simulink model "Quad_att_control"  (R2022b)
settings: Solver=ode4  StartTime=0.0  StopTime=100  FixedStep=0.001  RelTol=1e-3  EnableMultiTasking=on
model workspace (MAT data in the model file):
  A_m = [0  0  0  1  0  0; 0  0  0  0  1  0; 0  0  0  0  0  1; 0  0  0  0  1  1; 0  0  0  1  0  1; 0  0  0  1  1  0]
  A_r = [0  0  0  1  0  0; 0  0  0  0  1  0; 0  0  0  0  0  1; -1  0  0  -6  0  0; 0  -1  0  0  -6  0; 0  0  -1  0  0  -6]
  B_m = [0  0  0; 0  0  0; 0  0  0; 1  0  0; 0  1  0; 0  0  1]
  B_r = [0  0  0; 0  0  0; 0  0  0; 1  0  0; 0  1  0; 0  0  1]
  W_n = 2
  Zeta = 1.5
undefined symbols (not defined in the file): d2r, params, r2d
libraries: slpidlib x3, sharedtransform x2, matrix_library x2, sharedutil x2, uavutilslib x2, slctrlblks x1
settings Model: SimulationMode=accelerator  ParameterArgumentNames=A_r,Zeta  Creator=dsai9  LastModifiedBy=dsai9
settings SolverCC: PositivePriorityOrder=on
settings OptimizationCC: EnhancedBackFolding=on  PassReuseOutputArgsAs=Individual arguments  ZeroExternalMemoryAtStartup=off  ZeroInternalMemoryAtStartup=off  MaxStackSize=64  OptimizeBlockOrder=speed  DifferentSizesBufferReuse=on  OptimizationCustomize=off  EfficientTunableParamExpr=on
settings DebuggingCC: ParameterTunabilityLossMsg=error
settings HardwareCC: ProdBitPerPointer=32  ProdBitPerSizeT=32  ProdBitPerPtrDiffT=32  ProdLargestAtomicInteger=Long  ProdLargestAtomicFloat=Double  ProdWordSize=32  ProdLongLongMode=on  ProdHWDeviceType=ARM Compatible->ARM Cortex
settings RTWCC: Description=Embedded Coder  SystemTargetFile=ert.tlc  HardwareBoard=Raspberry Pi  TLCOptions="-aInlineSetEventsForThisBaseRateFcn=TLC_FALSE -aSuppressMultiTaskScheduler=TLC_FALSE  -aRateBasedStepFcn=0"  TemplateMakefile=ert_default_tmf  Toolchain=GNU GCC Embedded Linux  BuildConfiguration=Faster Runs
settings CodeAppCC: ForceParamTrailComments=on  IgnoreCustomStorageClasses=off  OperatorAnnotations=on  SimulinkDataObjDesc=on  SFDataObjDesc=on  InsertBlockDesc=on
settings ERTTargetCC: SupportVariableSizeSignals=on  ExtModeTransport=2  ExtModeStaticAlloc=on  ExtModeMexFile=ext_xcp  ExtModeIntrfLevel=Level2 - Open

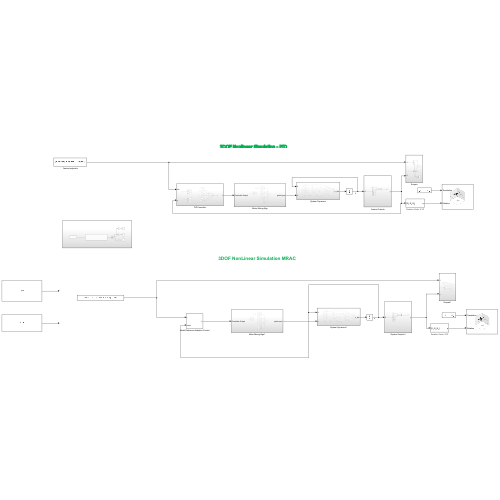
[thumbnail: Simulink's stored preview of the top-level diagram]
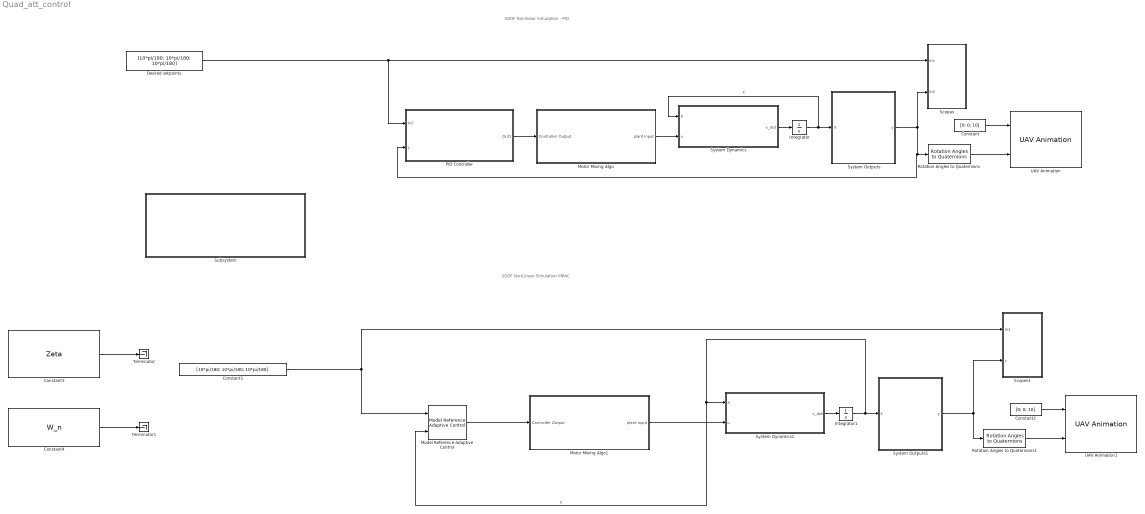
== system Quad_att_control ==
  note: 3DOF NonLinear Simulation MRAC
  note: 3DOF Nonlinear Simulation - PID
  Constant : Constant  Value=[0; 0; 10]
  Constant1 : Constant  Value=[10*pi/180; 10*pi/180; 10*pi/180]
  Constant2 : Constant  Value=[0; 0; 10]
  Constant3 : Constant  Value=Zeta
  Constant4 : Constant  Value=W_n
  Desired setpoints : Constant  Value=[10*pi/180; 10*pi/180; 10*pi/180]
  Integrator : Integrator  InitialCondition=[0;0;0;0;0;0]
  Integrator1 : Integrator  InitialCondition=[0;0;0;0;0;0]
  Model Reference Adaptive Control : slctrlblks/Model Reference Adaptive Control  selectType=Direct  A=A_m  B=B_m  Ahat=0  ALrEnable=on  gamma_a=1  ALrEnableMod=on  Bhat=1  BLrEnable=on  gamma_b=1  BLrEnableMod=on  externalKtauEnable=off  k_tau=-1  estParamOutput=off  Am=A_r  Bm=B_r  kx=0  FBLrEnable=on  gamma_kx=200  FBLrEnableMod=off  kr=0  FFLrEnable=on  gamma_kr=200  FFLrEnableMod=off  AdaptEnable=off  gamma=1  WLrEnableMod=on  Q=1  FeatureTypeOptions=State  nCen=20  cSpanMin=-1  cSpanMax=1  cSig=5  adaptiveCntrlOutport=off  modChoice=None  sigma_val=0.1
  Motor Mixing Algo : Subsystem
  Motor Mixing Algo1 : Subsystem
  PID Controller : Subsystem
  Rotation Angles to Quaternions : sharedtransform/Rotation Angles to Quaternions  rotationOrder=XYZ  aMode=aMode
  Rotation Angles to Quaternions1 : sharedtransform/Rotation Angles to Quaternions  rotationOrder=XYZ  aMode=aMode
  Scopes : Subsystem
  Scopes1 : Subsystem
  Subsystem : Subsystem
  System Dynamics : Subsystem
  System Dynamics1 : Subsystem
  System Outputs : Subsystem
  System Outputs1 : Subsystem
  Terminator : Terminator
  Terminator1 : Terminator
  UAV Animation : uavutilslib/UAV Animation  UAVType=Multirotor  UAVSize=1  InertialZDirection=Down  SampleTime=-1
  UAV Animation1 : uavutilslib/UAV Animation  UAVType=Multirotor  UAVSize=1  InertialZDirection=Down  SampleTime=-1
  wires:
  System Dynamics/1(x_dot) -> Integrator/1
  Integrator/1 -> System Dynamics/1(X), System Outputs/1(X)  "X"
  Motor Mixing Algo/1(plant input) -> System Dynamics/2(u)
  PID Controller/1(Out1) -> Motor Mixing Algo/1(Controller Output)
  System Outputs/1(y) -> Scopes/2(In2), Rotation Angles to Quaternions/1, PID Controller/2(y)
  Desired setpoints/1 -> PID Controller/1(Xd), Scopes/1(In1)
  Constant/1 -> UAV Animation/1
  Rotation Angles to Quaternions/1 -> UAV Animation/2
  Motor Mixing Algo1/1(plant input) -> System Dynamics1/2(u)
  System Dynamics1/1(x_dot) -> Integrator1/1
  Integrator1/1 -> System Outputs1/1(X), System Dynamics1/1(X), Model Reference Adaptive Control/2  "X"
  Model Reference Adaptive Control/1 -> Motor Mixing Algo1/1(Controller Output)
  Constant1/1 -> Model Reference Adaptive Control/1, Scopes1/1(In1)
  System Outputs1/1(y) -> Rotation Angles to Quaternions1/1, Scopes1/2(y)
  Rotation Angles to Quaternions1/1 -> UAV Animation1/2
  Constant2/1 -> UAV Animation1/1
  Constant3/1 -> Terminator/1
  Constant4/1 -> Terminator1/1

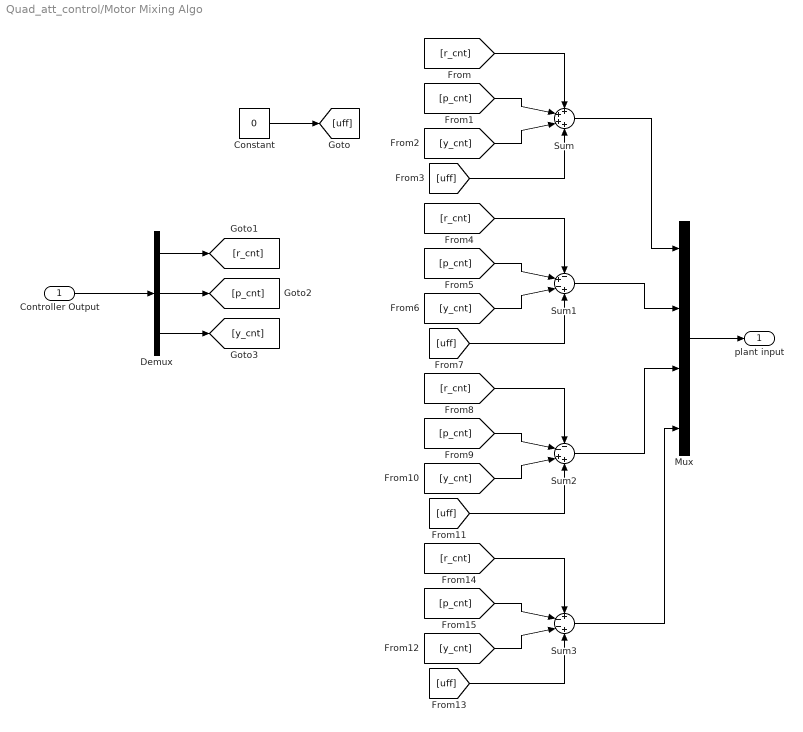
== system Quad_att_control/Motor Mixing Algo ==
  Controller Output : Inport
  Constant : Constant  Value=0
  Demux : Demux  Outputs=3
  Mux : Mux
  Sum : Sum  Inputs=++++
  Sum1 : Sum  Inputs=-+-+
  Sum2 : Sum  Inputs=--++
  Sum3 : Sum  Inputs=+--+
  plant input : Outport
  wires:
  Constant/1 -> [uff]
  Controller Output/1 -> Demux/1
  Demux/1 -> [r_cnt]
  Demux/3 -> [y_cnt]
  Demux/2 -> [p_cnt]
  Mux/1 -> plant input/1
  [r_cnt] -> Sum/1
  [p_cnt] -> Sum/2
  [y_cnt] -> Sum/3
  [uff] -> Sum/4
  Sum/1 -> Mux/1
  Sum1/1 -> Mux/2
  [uff] -> Sum1/4
  [y_cnt] -> Sum1/3
  [p_cnt] -> Sum1/2
  [r_cnt] -> Sum1/1
  [r_cnt] -> Sum2/1
  [p_cnt] -> Sum2/2
  [y_cnt] -> Sum2/3
  [uff] -> Sum2/4
  Sum2/1 -> Mux/3
  Sum3/1 -> Mux/4
  [uff] -> Sum3/4
  [y_cnt] -> Sum3/3
  [p_cnt] -> Sum3/2
  [r_cnt] -> Sum3/1

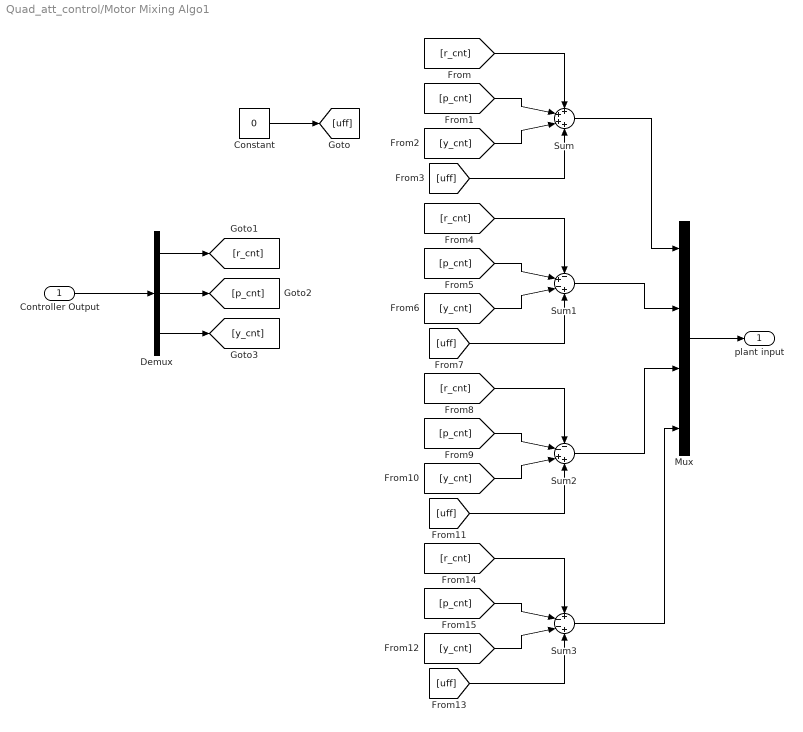
== system Quad_att_control/Motor Mixing Algo1 ==
  Controller Output : Inport
  Constant : Constant  Value=0
  Demux : Demux  Outputs=3
  Mux : Mux
  Sum : Sum  Inputs=++++
  Sum1 : Sum  Inputs=-+-+
  Sum2 : Sum  Inputs=--++
  Sum3 : Sum  Inputs=+--+
  plant input : Outport
  wires:
  [r_cnt] -> Sum3/1
  [p_cnt] -> Sum3/2
  [y_cnt] -> Sum3/3
  [uff] -> Sum3/4
  Sum3/1 -> Mux/4
  Sum2/1 -> Mux/3
  [uff] -> Sum2/4
  [y_cnt] -> Sum2/3
  [p_cnt] -> Sum2/2
  [r_cnt] -> Sum2/1
  [r_cnt] -> Sum1/1
  [p_cnt] -> Sum1/2
  [y_cnt] -> Sum1/3
  [uff] -> Sum1/4
  Sum1/1 -> Mux/2
  Sum/1 -> Mux/1
  [uff] -> Sum/4
  [y_cnt] -> Sum/3
  [p_cnt] -> Sum/2
  [r_cnt] -> Sum/1
  Mux/1 -> plant input/1
  Demux/2 -> [p_cnt]
  Demux/3 -> [y_cnt]
  Demux/1 -> [r_cnt]
  Controller Output/1 -> Demux/1
  Constant/1 -> [uff]

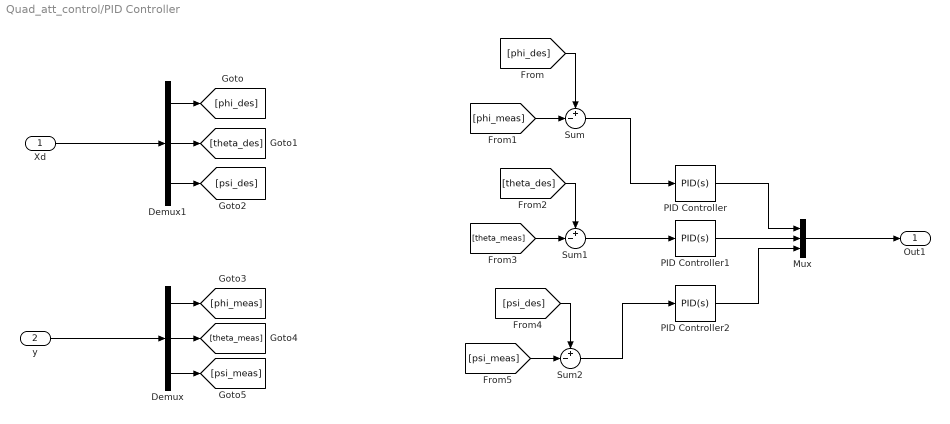
== system Quad_att_control/PID Controller ==
  Xd : Inport
  y : Inport  Port=2
  Demux : Demux  Outputs=3
  Demux1 : Demux  Outputs=3
  Mux : Mux  Inputs=3
  PID Controller : slpidlib/PID Controller  Controller=PID  Form=Parallel  TimeDomain=Continuous-time  UseExternalTs=off  SampleTime=-1  IntegratorMethod=Forward Euler  FilterMethod=Forward Euler  ControllerParametersSource=internal  P=100  I=0  UseKiTs=off  D=300  N=1  UseFilter=on  TunerSelectOption=Transfer Function Based (PID Tuner App)  InitialConditionSource=internal  InitialConditionForIntegrator=0  InitialConditionForFilter=0  DifferentiatorICPrevScaledInput=0  ExternalReset=none  TrackingMode=off  Kt=1  LimitOutput=off  SatLimitsSource=internal  UpperSaturationLimit=inf  LowerSaturationLimit=-inf  LinearizeAsGain=on  AntiWindupMode=none  Kb=1  LimitIntegrator=off  UpperIntegratorSaturationLimit=inf  LowerIntegratorSaturationLimit=-inf  POutMin=[]  POutMax=[]  IOutMin=[]  IOutMax=[]  DOutMin=[]  DOutMax=[]  NOutMin=[]  NOutMax=[]  SumOutMin=[]  SumOutMax=[]  SaturationOutMin=[]  SaturationOutMax=[]  PParamMin=[]  PParamMax=[]  IParamMin=[]  IParamMax=[]  DParamMin=[]  DParamMax=[]  NParamMin=[]  NParamMax=[]  KbParamMin=[]  KbParamMax=[]  KtParamMin=[]  KtParamMax=[]  KbOutMin=[]  KbOutMax=[]  KtOutMin=[]  KtOutMax=[]  IntegratorOutMin=[]  IntegratorOutMax=[]  FilterOutMin=[]  FilterOutMax=[]  SumI1OutMin=[]  SumI1OutMax=[]  SumI2OutMin=[]  SumI2OutMax=[]  SumI3OutMin=[]  SumI3OutMax=[]  SumI4OutMin=[]  SumI4OutMax=[]  SumDOutMin=[]  SumDOutMax=[]  DifferentiatorOutMin=[]  DifferentiatorOutMax=[]  FilterDiffOutCoefMin=[]  FilterDiffOutCoefMax=[]  ReciprocalOutMin=[]  ReciprocalOutMax=[]  SumDenOutMin=[]  SumDenOutMax=[]  SumNumOutMin=[]  SumNumOutMax=[]  DivideOutMin=[]  DivideOutMax=[]  UdiffTsProdOutMin=[]  UdiffTsProdOutMax=[]  NTsProdOutMin=[]  NTsProdOutMax=[]  UintegralTsProdOutMin=[]  UintegralTsProdOutMax=[]  UngainTsProdOutMin=[]  UngainTsProdOutMax=[]  ClampingZeroOutDataTypeStr=Inherit: Inherit via back propagation  ClampingZeroOutMin=[]  ClampingZeroOutMax=[]  FilterDenConstantOutDataTypeStr=Inherit: Inherit via back propagation  FilterDenConstantOutMin=[]  FilterDenConstantOutMax=[]  PCopyOutDataTypeStr=Inherit: Inherit via back propagation  PCopyOutMin=[]  PCopyOutMax=[]  NCopyOutDataTypeStr=Inherit: Inherit via back propagation  NCopyOutMin=[]  NCopyOutMax=[]  IntegratorContinuousStateAttributes=''  IntegratorStateMustResolveToSignalObject=off  IntegratorRTWStateStorageClass=Auto  FilterContinuousStateAttributes=''  FilterStateMustResolveToSignalObject=off  FilterRTWStateStorageClass=Auto  ParallelPVariant=InternalParameters  IdealPVariant=Disabled  IVariant=InternalParameters  DVariant=InternalParameters  IntegratorVariant=Continuous  SatVariant=Disabled  AWVariant=Passthrough  PCopyVariant=Disabled  TRVariant=Disabled  FdbkBlocksVariant=Forward  IdealPFdbkVariant=Disabled  SatFdbkVariant=Disabled  DerivativeFilterVariant=ContFilter  NVariant=InternalParameters  NCopyVariant=Disabled  FilterICVariant=InternalICsFilter  IntegratorICVariant=InternalICs  ExternalResetVariant=Disabled  TRSumVariant=Passthrough  SumFdbkVariant=Disabled  SumVariant=Sum_PID  TsampFilterVariant=InternalTs  TsampNgainVariant=Passthrough  TsampIntegralVariant=Passthrough  ExternalSaturationOutDataTypeStr=Inherit: Same as second input
  PID Controller1 : slpidlib/PID Controller  Controller=PID  Form=Parallel  TimeDomain=Continuous-time  UseExternalTs=off  SampleTime=-1  IntegratorMethod=Forward Euler  FilterMethod=Forward Euler  ControllerParametersSource=internal  P=100  I=0  UseKiTs=off  D=300  N=1  UseFilter=on  TunerSelectOption=Transfer Function Based (PID Tuner App)  InitialConditionSource=internal  InitialConditionForIntegrator=0  InitialConditionForFilter=0  DifferentiatorICPrevScaledInput=0  ExternalReset=none  TrackingMode=off  Kt=1  LimitOutput=off  SatLimitsSource=internal  UpperSaturationLimit=inf  LowerSaturationLimit=-inf  LinearizeAsGain=on  AntiWindupMode=none  Kb=1  LimitIntegrator=off  UpperIntegratorSaturationLimit=inf  LowerIntegratorSaturationLimit=-inf  POutMin=[]  POutMax=[]  IOutMin=[]  IOutMax=[]  DOutMin=[]  DOutMax=[]  NOutMin=[]  NOutMax=[]  SumOutMin=[]  SumOutMax=[]  SaturationOutMin=[]  SaturationOutMax=[]  PParamMin=[]  PParamMax=[]  IParamMin=[]  IParamMax=[]  DParamMin=[]  DParamMax=[]  NParamMin=[]  NParamMax=[]  KbParamMin=[]  KbParamMax=[]  KtParamMin=[]  KtParamMax=[]  KbOutMin=[]  KbOutMax=[]  KtOutMin=[]  KtOutMax=[]  IntegratorOutMin=[]  IntegratorOutMax=[]  FilterOutMin=[]  FilterOutMax=[]  SumI1OutMin=[]  SumI1OutMax=[]  SumI2OutMin=[]  SumI2OutMax=[]  SumI3OutMin=[]  SumI3OutMax=[]  SumI4OutMin=[]  SumI4OutMax=[]  SumDOutMin=[]  SumDOutMax=[]  DifferentiatorOutMin=[]  DifferentiatorOutMax=[]  FilterDiffOutCoefMin=[]  FilterDiffOutCoefMax=[]  ReciprocalOutMin=[]  ReciprocalOutMax=[]  SumDenOutMin=[]  SumDenOutMax=[]  SumNumOutMin=[]  SumNumOutMax=[]  DivideOutMin=[]  DivideOutMax=[]  UdiffTsProdOutMin=[]  UdiffTsProdOutMax=[]  NTsProdOutMin=[]  NTsProdOutMax=[]  UintegralTsProdOutMin=[]  UintegralTsProdOutMax=[]  UngainTsProdOutMin=[]  UngainTsProdOutMax=[]  ClampingZeroOutDataTypeStr=Inherit: Inherit via back propagation  ClampingZeroOutMin=[]  ClampingZeroOutMax=[]  FilterDenConstantOutDataTypeStr=Inherit: Inherit via back propagation  FilterDenConstantOutMin=[]  FilterDenConstantOutMax=[]  PCopyOutDataTypeStr=Inherit: Inherit via back propagation  PCopyOutMin=[]  PCopyOutMax=[]  NCopyOutDataTypeStr=Inherit: Inherit via back propagation  NCopyOutMin=[]  NCopyOutMax=[]  IntegratorContinuousStateAttributes=''  IntegratorStateMustResolveToSignalObject=off  IntegratorRTWStateStorageClass=Auto  FilterContinuousStateAttributes=''  FilterStateMustResolveToSignalObject=off  FilterRTWStateStorageClass=Auto  ParallelPVariant=InternalParameters  IdealPVariant=Disabled  IVariant=InternalParameters  DVariant=InternalParameters  IntegratorVariant=Continuous  SatVariant=Disabled  AWVariant=Passthrough  PCopyVariant=Disabled  TRVariant=Disabled  FdbkBlocksVariant=Forward  IdealPFdbkVariant=Disabled  SatFdbkVariant=Disabled  DerivativeFilterVariant=ContFilter  NVariant=InternalParameters  NCopyVariant=Disabled  FilterICVariant=InternalICsFilter  IntegratorICVariant=InternalICs  ExternalResetVariant=Disabled  TRSumVariant=Passthrough  SumFdbkVariant=Disabled  SumVariant=Sum_PID  TsampFilterVariant=InternalTs  TsampNgainVariant=Passthrough  TsampIntegralVariant=Passthrough  ExternalSaturationOutDataTypeStr=Inherit: Same as second input
  PID Controller2 : slpidlib/PID Controller  Controller=PID  Form=Parallel  TimeDomain=Continuous-time  UseExternalTs=off  SampleTime=-1  IntegratorMethod=Forward Euler  FilterMethod=Forward Euler  ControllerParametersSource=internal  P=500  I=0  UseKiTs=off  D=1000  N=1  UseFilter=on  TunerSelectOption=Transfer Function Based (PID Tuner App)  InitialConditionSource=internal  InitialConditionForIntegrator=0  InitialConditionForFilter=0  DifferentiatorICPrevScaledInput=0  ExternalReset=none  TrackingMode=off  Kt=1  LimitOutput=off  SatLimitsSource=internal  UpperSaturationLimit=inf  LowerSaturationLimit=-inf  LinearizeAsGain=on  AntiWindupMode=none  Kb=1  LimitIntegrator=off  UpperIntegratorSaturationLimit=inf  LowerIntegratorSaturationLimit=-inf  POutMin=[]  POutMax=[]  IOutMin=[]  IOutMax=[]  DOutMin=[]  DOutMax=[]  NOutMin=[]  NOutMax=[]  SumOutMin=[]  SumOutMax=[]  SaturationOutMin=[]  SaturationOutMax=[]  PParamMin=[]  PParamMax=[]  IParamMin=[]  IParamMax=[]  DParamMin=[]  DParamMax=[]  NParamMin=[]  NParamMax=[]  KbParamMin=[]  KbParamMax=[]  KtParamMin=[]  KtParamMax=[]  KbOutMin=[]  KbOutMax=[]  KtOutMin=[]  KtOutMax=[]  IntegratorOutMin=[]  IntegratorOutMax=[]  FilterOutMin=[]  FilterOutMax=[]  SumI1OutMin=[]  SumI1OutMax=[]  SumI2OutMin=[]  SumI2OutMax=[]  SumI3OutMin=[]  SumI3OutMax=[]  SumI4OutMin=[]  SumI4OutMax=[]  SumDOutMin=[]  SumDOutMax=[]  DifferentiatorOutMin=[]  DifferentiatorOutMax=[]  FilterDiffOutCoefMin=[]  FilterDiffOutCoefMax=[]  ReciprocalOutMin=[]  ReciprocalOutMax=[]  SumDenOutMin=[]  SumDenOutMax=[]  SumNumOutMin=[]  SumNumOutMax=[]  DivideOutMin=[]  DivideOutMax=[]  UdiffTsProdOutMin=[]  UdiffTsProdOutMax=[]  NTsProdOutMin=[]  NTsProdOutMax=[]  UintegralTsProdOutMin=[]  UintegralTsProdOutMax=[]  UngainTsProdOutMin=[]  UngainTsProdOutMax=[]  ClampingZeroOutDataTypeStr=Inherit: Inherit via back propagation  ClampingZeroOutMin=[]  ClampingZeroOutMax=[]  FilterDenConstantOutDataTypeStr=Inherit: Inherit via back propagation  FilterDenConstantOutMin=[]  FilterDenConstantOutMax=[]  PCopyOutDataTypeStr=Inherit: Inherit via back propagation  PCopyOutMin=[]  PCopyOutMax=[]  NCopyOutDataTypeStr=Inherit: Inherit via back propagation  NCopyOutMin=[]  NCopyOutMax=[]  IntegratorContinuousStateAttributes=''  IntegratorStateMustResolveToSignalObject=off  IntegratorRTWStateStorageClass=Auto  FilterContinuousStateAttributes=''  FilterStateMustResolveToSignalObject=off  FilterRTWStateStorageClass=Auto  ParallelPVariant=InternalParameters  IdealPVariant=Disabled  IVariant=InternalParameters  DVariant=InternalParameters  IntegratorVariant=Continuous  SatVariant=Disabled  AWVariant=Passthrough  PCopyVariant=Disabled  TRVariant=Disabled  FdbkBlocksVariant=Forward  IdealPFdbkVariant=Disabled  SatFdbkVariant=Disabled  DerivativeFilterVariant=ContFilter  NVariant=InternalParameters  NCopyVariant=Disabled  FilterICVariant=InternalICsFilter  IntegratorICVariant=InternalICs  ExternalResetVariant=Disabled  TRSumVariant=Passthrough  SumFdbkVariant=Disabled  SumVariant=Sum_PID  TsampFilterVariant=InternalTs  TsampNgainVariant=Passthrough  TsampIntegralVariant=Passthrough  ExternalSaturationOutDataTypeStr=Inherit: Same as second input
  Sum : Sum  Inputs=+-|
  Sum1 : Sum  Inputs=+-|
  Sum2 : Sum  Inputs=+-|
  Out1 : Outport
  wires:
  PID Controller2/1 -> Mux/3
  PID Controller/1 -> Mux/1
  PID Controller1/1 -> Mux/2
  Mux/1 -> Out1/1
  y/1 -> Demux/1
  Xd/1 -> Demux1/1
  Sum/1 -> PID Controller/1
  Demux1/1 -> [phi_des]
  Demux1/2 -> [theta_des]
  Demux1/3 -> [psi_des]
  Demux/1 -> [phi_meas]
  Demux/2 -> [theta_meas]
  Demux/3 -> [psi_meas]
  [phi_des] -> Sum/1
  [phi_meas] -> Sum/2
  [theta_meas] -> Sum1/2
  [theta_des] -> Sum1/1
  Sum1/1 -> PID Controller1/1
  Sum2/1 -> PID Controller2/1
  [psi_des] -> Sum2/1
  [psi_meas] -> Sum2/2

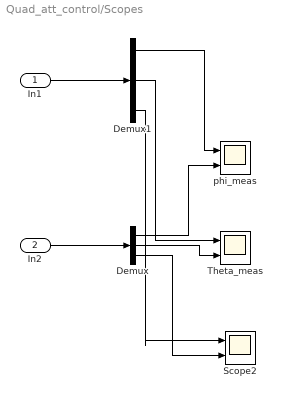
== system Quad_att_control/Scopes ==
  In1 : Inport
  In2 : Inport  Port=2
  Demux : Demux  Outputs=3
  Demux1 : Demux  Outputs=3
  Scope2 : Scope  NumInputPorts=2
  Theta_meas : Scope  NumInputPorts=2
  phi_meas : Scope  NumInputPorts=2
  wires:
  In1/1 -> Demux1/1
  Demux1/1 -> phi_meas/1
  Demux/3 -> Scope2/2
  Demux/1 -> phi_meas/2
  In2/1 -> Demux/1
  Demux/2 -> Theta_meas/2
  Demux1/3 -> Scope2/1
  Demux1/2 -> Theta_meas/1

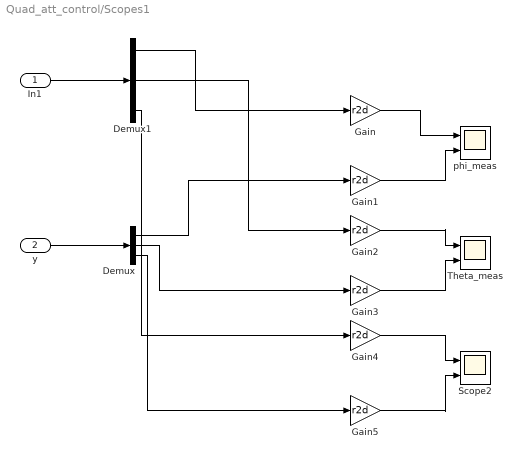
== system Quad_att_control/Scopes1 ==
  In1 : Inport
  y : Inport  Port=2
  Demux : Demux  Outputs=3
  Demux1 : Demux  Outputs=3
  Gain{,1..5} (6 alike) : Gain  Gain=r2d
  Scope2 : Scope  NumInputPorts=2
  Theta_meas : Scope  NumInputPorts=2
  phi_meas : Scope  NumInputPorts=2
  wires:
  Demux1/2 -> Gain2/1
  Demux1/3 -> Gain4/1
  Demux/2 -> Gain3/1
  y/1 -> Demux/1
  Demux/1 -> Gain1/1
  Demux/3 -> Gain5/1
  Demux1/1 -> Gain/1
  In1/1 -> Demux1/1
  Gain/1 -> phi_meas/1
  Gain1/1 -> phi_meas/2
  Gain2/1 -> Theta_meas/1
  Gain3/1 -> Theta_meas/2
  Gain4/1 -> Scope2/1
  Gain5/1 -> Scope2/2

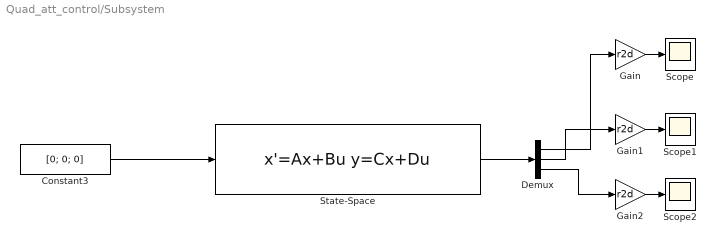
== system Quad_att_control/Subsystem ==
  Constant3 : Constant  Value=[0; 0; 0]
  Demux : Demux  Outputs=3
  Gain : Gain  Gain=r2d
  Gain1 : Gain  Gain=r2d
  Gain2 : Gain  Gain=r2d
  Scope : Scope
  Scope1 : Scope
  Scope2 : Scope
  State-Space : StateSpace  A=A_r  B=B_r  C=[1 0 0 0 0 0; 0 1 0 0 0 0; 0 0 1 0 0 0]  D=[0 0 0; 0 0 0; 0 0 0]  InitialCondition=[10*d2r; 10*d2r; 10*d2r; 0; 0; 0]  ParameterTunability=Unconstrained
  wires:
  Constant3/1 -> State-Space/1
  State-Space/1 -> Demux/1
  Demux/1 -> Gain/1
  Demux/2 -> Gain1/1
  Demux/3 -> Gain2/1
  Gain/1 -> Scope/1
  Gain1/1 -> Scope1/1
  Gain2/1 -> Scope2/1

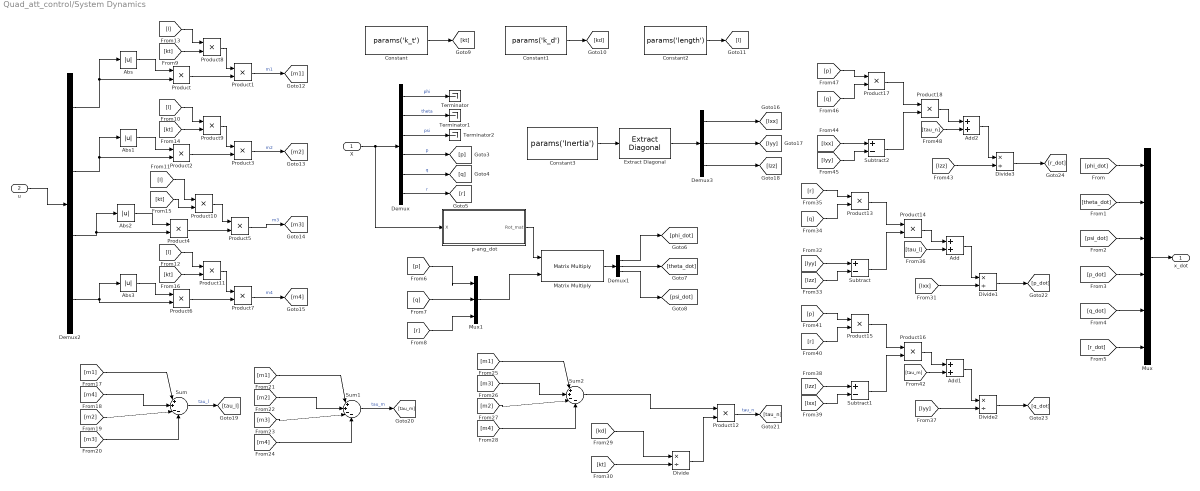
== system Quad_att_control/System Dynamics ==
  X : Inport
  u : Inport  Port=2
  Abs{,1..3} (4 alike) : Abs  SaturateOnIntegerOverflow=off
  Add : Sum
  Add1 : Sum
  Add2 : Sum
  Constant : Constant  Value=params('k_t')
  Constant1 : Constant  Value=params('k_d')
  Constant2 : Constant  Value=params('length')
  Constant3 : Constant  Value=params('Inertia')
  Demux : Demux  Outputs=6
  Demux1 : Demux  Outputs=3
  Demux2 : Demux
  Demux3 : Demux  Outputs=3
  Divide{,1..3} (4 alike) : Product  Inputs=*/
  Extract Diagonal : matrix_library/Extract Diagonal
      settings: LibrarySourceBlock=|
      | simulink/Matrix
      | Operations/Extract Diagonal
  Matrix Multiply : Product  Multiplication=Matrix(*)
  Mux : Mux  Inputs=6
  Mux1 : Mux  Inputs=3
  Product{,1..18} (19 alike) : Product
  Subtract : Sum  Inputs=+-
  Subtract1 : Sum  Inputs=+-
  Subtract2 : Sum  Inputs=+-
  Sum : Sum  Inputs=|++--
  Sum1 : Sum  Inputs=|++--
  Sum2 : Sum  Inputs=|++--
  Terminator : Terminator
  Terminator1 : Terminator
  Terminator2 : Terminator
  p-ang_dot : Subsystem
  x_dot : Outport
  wires:
  Demux/4 -> [p]  "p"
  Sum1/1 -> [tau_m]  "tau_m"
  [p] -> Product17/1
  [Ixx] -> Divide1/2
  Demux2/2 -> Abs1/1, Product2/2
  Demux1/1 -> [phi_dot]
  Demux3/2 -> [Iyy]
  X/1 -> p-ang_dot/1(X), Demux/1
  [tau_l] -> Add/2
  Demux2/1 -> Product/2, Abs/1
  [tau_n] -> Add2/2
  [kt] -> Product8/2
  Product12/1 -> [tau_n]  "tau_n"
  Divide3/1 -> [r_dot]
  Abs2/1 -> Product4/1
  [q] -> Product17/2
  Demux/1 -> Terminator/1  "phi"
  Constant1/1 -> [kd]
  Product11/1 -> Product7/1
  Product10/1 -> Product5/1
  [p_dot] -> Mux/4
  Product15/1 -> Product16/1
  Add2/1 -> Divide3/1
  [q_dot] -> Mux/5
  Sum/1 -> [tau_l]  "tau_l"
  [l] -> Product10/1
  Product17/1 -> Product18/1
  [m4] -> Sum/2
  Product8/1 -> Product1/1
  [p] -> Mux1/1
  [Izz] -> Divide3/2
  [m2] -> Sum/3
  [Ixx] -> Subtract2/1
  Demux/3 -> Terminator2/1  "psi"
  Product18/1 -> Add2/1
  Subtract2/1 -> Product18/2
  Product7/1 -> [m4]  "m4"
  [phi_dot] -> Mux/1
  [l] -> Product8/1
  [Iyy] -> Subtract2/2
  Demux/5 -> [q]  "q"
  [kt] -> Product11/2
  Product2/1 -> Product3/2
  Constant/1 -> [kt]
  [r] -> Mux1/3
  [m3] -> Sum/4
  Demux1/2 -> [theta_dot]
  [kt] -> Product10/2
  [m1] -> Sum/1
  Product/1 -> Product1/2
  p-ang_dot/1(Rot_mat) -> Matrix Multiply/1
  Divide1/1 -> [p_dot]
  Divide/1 -> Product12/2
  Product3/1 -> [m2]  "m2"
  Product16/1 -> Add1/1
  Mux1/1 -> Matrix Multiply/2
  Demux/2 -> Terminator1/1  "theta"
  [psi_dot] -> Mux/3
  [r_dot] -> Mux/6
  Demux1/3 -> [psi_dot]
  [theta_dot] -> Mux/2
  Abs1/1 -> Product2/1
  Subtract/1 -> Product14/2
  Demux/6 -> [r]  "r"
  Demux2/3 -> Product4/2, Abs2/1
  Product4/1 -> Product5/2
  [q] -> Mux1/2
  Constant2/1 -> [l]
  Matrix Multiply/1 -> Demux1/1
  Product14/1 -> Add/1
  Add/1 -> Divide1/1
  Divide2/1 -> [q_dot]
  Add1/1 -> Divide2/1
  [l] -> Product11/1
  [tau_m] -> Add1/2
  Subtract1/1 -> Product16/2
  [r] -> Product15/2
  [Ixx] -> Subtract1/2
  [Iyy] -> Divide2/2
  [Izz] -> Subtract1/1
  [p] -> Product15/1
  Extract Diagonal/1 -> Demux3/1
  [r] -> Product13/1
  Abs/1 -> Product/1
  Product6/1 -> Product7/2
  Demux2/4 -> Abs3/1, Product6/2
  Abs3/1 -> Product6/1
  Product1/1 -> [m1]  "m1"
  Demux3/3 -> [Izz]
  Constant3/1 -> Extract Diagonal/1
  [kd] -> Divide/1
  [kt] -> Product9/2
  Product9/1 -> Product3/1
  [l] -> Product9/1
  [m3] -> Sum1/3
  [m2] -> Sum1/2
  [m4] -> Sum1/4
  [m1] -> Sum1/1
  Product5/1 -> [m3]  "m3"
  u/1 -> Demux2/1
  [m1] -> Sum2/1
  [m3] -> Sum2/2
  [m2] -> Sum2/3
  [m4] -> Sum2/4
  Sum2/1 -> Product12/1
  Product13/1 -> Product14/1
  [q] -> Product13/2
  [kt] -> Divide/2
  [Iyy] -> Subtract/1
  [Izz] -> Subtract/2
  Demux3/1 -> [Ixx]
  Mux/1 -> x_dot/1

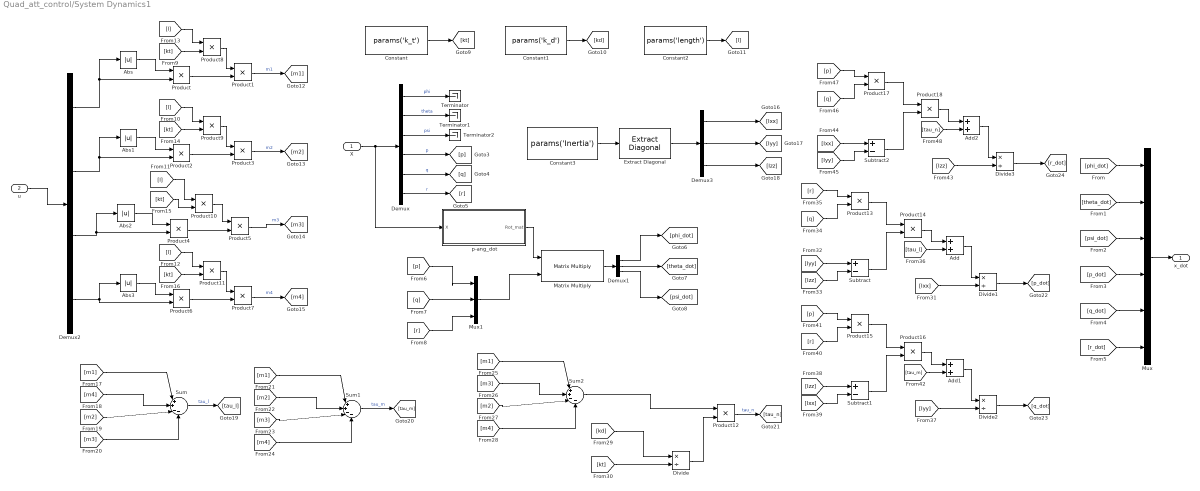
== system Quad_att_control/System Dynamics1 ==
  X : Inport
  u : Inport  Port=2
  Abs{,1..3} (4 alike) : Abs  SaturateOnIntegerOverflow=off
  Add : Sum
  Add1 : Sum
  Add2 : Sum
  Constant : Constant  Value=params('k_t')
  Constant1 : Constant  Value=params('k_d')
  Constant2 : Constant  Value=params('length')
  Constant3 : Constant  Value=params('Inertia')
  Demux : Demux  Outputs=6
  Demux1 : Demux  Outputs=3
  Demux2 : Demux
  Demux3 : Demux  Outputs=3
  Divide{,1..3} (4 alike) : Product  Inputs=*/
  Extract Diagonal : matrix_library/Extract Diagonal
      settings: LibrarySourceBlock=|
      | simulink/Matrix
      | Operations/Extract Diagonal
  Matrix Multiply : Product  Multiplication=Matrix(*)
  Mux : Mux  Inputs=6
  Mux1 : Mux  Inputs=3
  Product{,1..18} (19 alike) : Product
  Subtract : Sum  Inputs=+-
  Subtract1 : Sum  Inputs=+-
  Subtract2 : Sum  Inputs=+-
  Sum : Sum  Inputs=|++--
  Sum1 : Sum  Inputs=|++--
  Sum2 : Sum  Inputs=|++--
  Terminator : Terminator
  Terminator1 : Terminator
  Terminator2 : Terminator
  p-ang_dot : Subsystem
  x_dot : Outport
  wires:
  Mux/1 -> x_dot/1
  Demux3/1 -> [Ixx]
  [Izz] -> Subtract/2
  [Iyy] -> Subtract/1
  [kt] -> Divide/2
  [q] -> Product13/2
  Product13/1 -> Product14/1
  Sum2/1 -> Product12/1
  [m4] -> Sum2/4
  [m2] -> Sum2/3
  [m3] -> Sum2/2
  [m1] -> Sum2/1
  u/1 -> Demux2/1
  Product5/1 -> [m3]  "m3"
  [m1] -> Sum1/1
  [m4] -> Sum1/4
  [m2] -> Sum1/2
  [m3] -> Sum1/3
  [l] -> Product9/1
  Product9/1 -> Product3/1
  [kt] -> Product9/2
  [kd] -> Divide/1
  Constant3/1 -> Extract Diagonal/1
  Demux3/3 -> [Izz]
  Product1/1 -> [m1]  "m1"
  Abs3/1 -> Product6/1
  Demux2/4 -> Product6/2, Abs3/1
  Product6/1 -> Product7/2
  Abs/1 -> Product/1
  [r] -> Product13/1
  Extract Diagonal/1 -> Demux3/1
  [p] -> Product15/1
  [Izz] -> Subtract1/1
  [Iyy] -> Divide2/2
  [Ixx] -> Subtract1/2
  [r] -> Product15/2
  Subtract1/1 -> Product16/2
  [tau_m] -> Add1/2
  [l] -> Product11/1
  Add1/1 -> Divide2/1
  Divide2/1 -> [q_dot]
  Add/1 -> Divide1/1
  Product14/1 -> Add/1
  Matrix Multiply/1 -> Demux1/1
  Constant2/1 -> [l]
  [q] -> Mux1/2
  Product4/1 -> Product5/2
  Demux2/3 -> Abs2/1, Product4/2
  Demux/6 -> [r]  "r"
  Subtract/1 -> Product14/2
  Abs1/1 -> Product2/1
  [theta_dot] -> Mux/2
  Demux1/3 -> [psi_dot]
  [r_dot] -> Mux/6
  [psi_dot] -> Mux/3
  Demux/2 -> Terminator1/1  "theta"
  Mux1/1 -> Matrix Multiply/2
  Product16/1 -> Add1/1
  Product3/1 -> [m2]  "m2"
  Divide/1 -> Product12/2
  Divide1/1 -> [p_dot]
  p-ang_dot/1(Rot_mat) -> Matrix Multiply/1
  Product/1 -> Product1/2
  [m1] -> Sum/1
  [kt] -> Product10/2
  Demux1/2 -> [theta_dot]
  [m3] -> Sum/4
  [r] -> Mux1/3
  Constant/1 -> [kt]
  Product2/1 -> Product3/2
  [kt] -> Product11/2
  Demux/5 -> [q]  "q"
  [Iyy] -> Subtract2/2
  [l] -> Product8/1
  [phi_dot] -> Mux/1
  Product7/1 -> [m4]  "m4"
  Subtract2/1 -> Product18/2
  Product18/1 -> Add2/1
  Demux/3 -> Terminator2/1  "psi"
  [Ixx] -> Subtract2/1
  [m2] -> Sum/3
  [Izz] -> Divide3/2
  [p] -> Mux1/1
  Product8/1 -> Product1/1
  [m4] -> Sum/2
  Product17/1 -> Product18/1
  [l] -> Product10/1
  Sum/1 -> [tau_l]  "tau_l"
  [q_dot] -> Mux/5
  Add2/1 -> Divide3/1
  Product15/1 -> Product16/1
  [p_dot] -> Mux/4
  Product10/1 -> Product5/1
  Product11/1 -> Product7/1
  Constant1/1 -> [kd]
  Demux/1 -> Terminator/1  "phi"
  [q] -> Product17/2
  Abs2/1 -> Product4/1
  Divide3/1 -> [r_dot]
  Product12/1 -> [tau_n]  "tau_n"
  [kt] -> Product8/2
  [tau_n] -> Add2/2
  Demux2/1 -> Abs/1, Product/2
  [tau_l] -> Add/2
  X/1 -> Demux/1, p-ang_dot/1(X)
  Demux3/2 -> [Iyy]
  Demux1/1 -> [phi_dot]
  Demux2/2 -> Product2/2, Abs1/1
  [Ixx] -> Divide1/2
  [p] -> Product17/1
  Sum1/1 -> [tau_m]  "tau_m"
  Demux/4 -> [p]  "p"

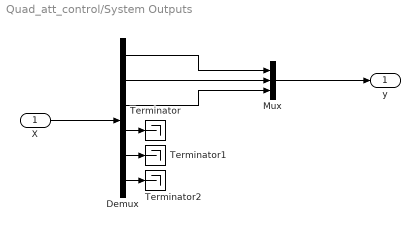
== system Quad_att_control/System Outputs ==
  X : Inport
  Demux : Demux  Outputs=6
  Mux : Mux  Inputs=3
  Terminator : Terminator
  Terminator1 : Terminator
  Terminator2 : Terminator
  y : Outport
  wires:
  Demux/6 -> Terminator2/1
  Demux/4 -> Terminator/1
  Demux/5 -> Terminator1/1
  X/1 -> Demux/1
  Demux/1 -> Mux/1
  Demux/2 -> Mux/2
  Demux/3 -> Mux/3
  Mux/1 -> y/1

== system Quad_att_control/System Outputs1 ==
  X : Inport
  Demux : Demux  Outputs=6
  Mux : Mux  Inputs=3
  Terminator : Terminator
  Terminator1 : Terminator
  Terminator2 : Terminator
  y : Outport
  wires:
  Mux/1 -> y/1
  Demux/3 -> Mux/3
  Demux/2 -> Mux/2
  Demux/1 -> Mux/1
  X/1 -> Demux/1
  Demux/5 -> Terminator1/1
  Demux/4 -> Terminator/1
  Demux/6 -> Terminator2/1

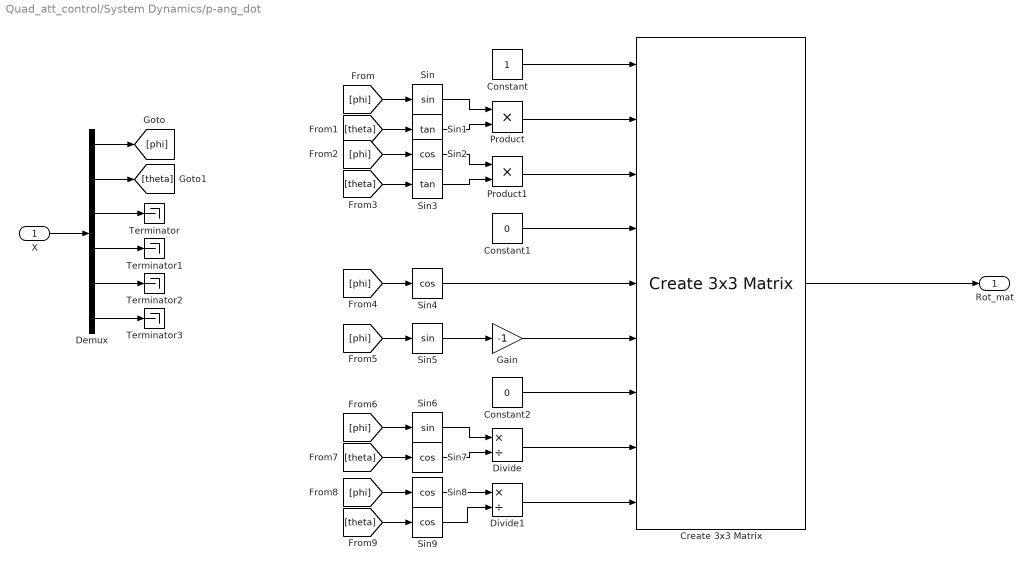
== system Quad_att_control/System Dynamics/p-ang_dot ==
  X : Inport
  Constant : Constant
  Constant1 : Constant  Value=0
  Constant2 : Constant  Value=0
  Create 3x3 Matrix : sharedutil/Create 3x3 Matrix  aMode=aMode
      settings: LibrarySourceBlock=aerolibutil/Create 3x3 Matrix
  Demux : Demux  Outputs=6
  Divide : Product  Inputs=*/  RndMeth=Zero  SaturateOnIntegerOverflow=on
  Divide1 : Product  Inputs=*/  RndMeth=Zero  SaturateOnIntegerOverflow=on
  Gain : Gain  Gain=-1
  Product : Product
  Product1 : Product
  Sin : Trigonometry
  Sin1 : Trigonometry  Operator=tan
  Sin{2,4,7..9} (5 alike) : Trigonometry  Operator=cos
  Sin3 : Trigonometry  Operator=tan
  Sin5 : Trigonometry
  Sin6 : Trigonometry
  Terminator{,1..3} (4 alike) : Terminator
  Rot_mat : Outport
  wires:
  Sin6/1 -> Divide/1
  [phi] -> Sin6/1
  Sin1/1 -> Product/2
  [theta] -> Sin7/1
  Constant2/1 -> Create 3x3 Matrix/7
  Constant/1 -> Create 3x3 Matrix/1
  [theta] -> Sin9/1
  Constant1/1 -> Create 3x3 Matrix/4
  Sin5/1 -> Gain/1
  Sin/1 -> Product/1
  Sin7/1 -> Divide/2
  [phi] -> Sin5/1
  [theta] -> Sin1/1
  Sin8/1 -> Divide1/1
  Gain/1 -> Create 3x3 Matrix/6
  Product/1 -> Create 3x3 Matrix/2
  [phi] -> Sin2/1
  Sin3/1 -> Product1/2
  Sin2/1 -> Product1/1
  Product1/1 -> Create 3x3 Matrix/3
  Divide1/1 -> Create 3x3 Matrix/9
  [theta] -> Sin3/1
  [phi] -> Sin4/1
  [phi] -> Sin/1
  Sin4/1 -> Create 3x3 Matrix/5
  Divide/1 -> Create 3x3 Matrix/8
  [phi] -> Sin8/1
  Sin9/1 -> Divide1/2
  Create 3x3 Matrix/1 -> Rot_mat/1
  X/1 -> Demux/1
  Demux/1 -> [phi]
  Demux/2 -> [theta]
  Demux/3 -> Terminator/1
  Demux/4 -> Terminator1/1
  Demux/5 -> Terminator2/1
  Demux/6 -> Terminator3/1

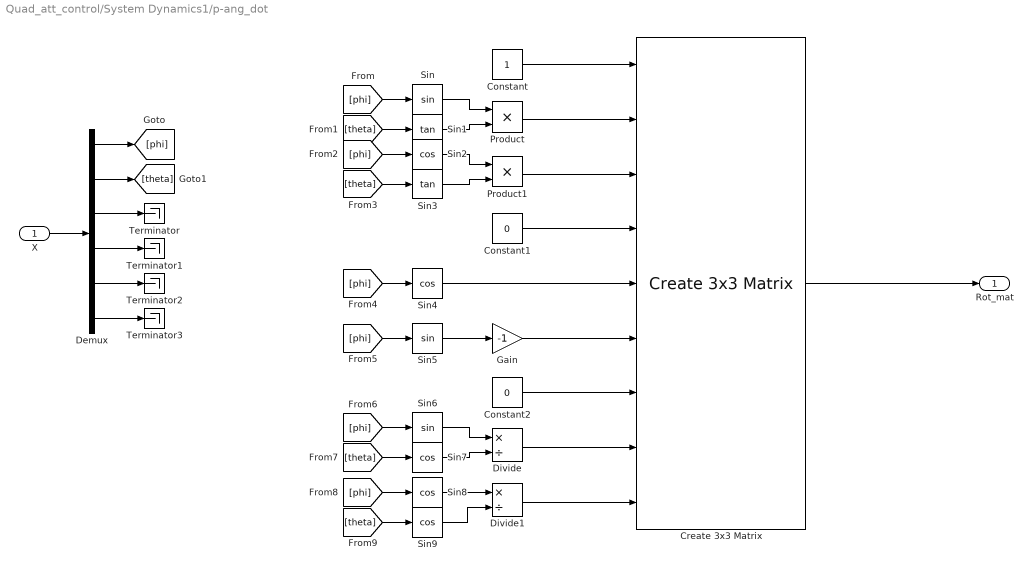
== system Quad_att_control/System Dynamics1/p-ang_dot ==
  X : Inport
  Constant : Constant
  Constant1 : Constant  Value=0
  Constant2 : Constant  Value=0
  Create 3x3 Matrix : sharedutil/Create 3x3 Matrix  aMode=aMode
      settings: LibrarySourceBlock=aerolibutil/Create 3x3 Matrix
  Demux : Demux  Outputs=6
  Divide : Product  Inputs=*/  RndMeth=Zero  SaturateOnIntegerOverflow=on
  Divide1 : Product  Inputs=*/  RndMeth=Zero  SaturateOnIntegerOverflow=on
  Gain : Gain  Gain=-1
  Product : Product
  Product1 : Product
  Sin : Trigonometry
  Sin1 : Trigonometry  Operator=tan
  Sin{2,4,7..9} (5 alike) : Trigonometry  Operator=cos
  Sin3 : Trigonometry  Operator=tan
  Sin5 : Trigonometry
  Sin6 : Trigonometry
  Terminator{,1..3} (4 alike) : Terminator
  Rot_mat : Outport
  wires:
  Demux/6 -> Terminator3/1
  Demux/5 -> Terminator2/1
  Demux/4 -> Terminator1/1
  Demux/3 -> Terminator/1
  Demux/2 -> [theta]
  Demux/1 -> [phi]
  X/1 -> Demux/1
  Create 3x3 Matrix/1 -> Rot_mat/1
  Sin9/1 -> Divide1/2
  [phi] -> Sin8/1
  Divide/1 -> Create 3x3 Matrix/8
  Sin4/1 -> Create 3x3 Matrix/5
  [phi] -> Sin/1
  [phi] -> Sin4/1
  [theta] -> Sin3/1
  Divide1/1 -> Create 3x3 Matrix/9
  Product1/1 -> Create 3x3 Matrix/3
  Sin2/1 -> Product1/1
  Sin3/1 -> Product1/2
  [phi] -> Sin2/1
  Product/1 -> Create 3x3 Matrix/2
  Gain/1 -> Create 3x3 Matrix/6
  Sin8/1 -> Divide1/1
  [theta] -> Sin1/1
  [phi] -> Sin5/1
  Sin7/1 -> Divide/2
  Sin/1 -> Product/1
  Sin5/1 -> Gain/1
  Constant1/1 -> Create 3x3 Matrix/4
  [theta] -> Sin9/1
  Constant/1 -> Create 3x3 Matrix/1
  Constant2/1 -> Create 3x3 Matrix/7
  [theta] -> Sin7/1
  Sin1/1 -> Product/2
  [phi] -> Sin6/1
  Sin6/1 -> Divide/1
